simulink model "Simulink_Test_Model"  (R2018a)
settings: Solver=ode15s  StartTime=0.0  StopTime=100  FixedStep=0.0001  RelTol=1e-3  EnableMultiTasking=on
libraries: simulink x1
settings Model: Creator=user  LastModifiedBy=user
settings SolverCC: ConcurrentTasks=on  AutoInsertRateTranBlk=on
settings DataIOCC: SaveFormat=StructureWithTime  SaveState=on  SignalLoggingName=logsOut
settings OptimizationCC: BlockReduction=off  BooleanDataType=off  OptimizeBlockIOStorage=off  BufferReuse=off  GlobalBufferReuse=off  ExpressionFolding=off  LocalBlockOutputs=off  InitFltsAndDblsToZero=on  OptimizeDataStoreBuffers=off  BusAssignmentInplaceUpdate=off
settings DebuggingCC: SaveWithParameterizedLinksMsg=none  UnderspecifiedInitializationDetection=Classic  MergeDetectMultiDrivingBlocksExec=none  CheckExecutionContextPreStartOutputMsg=on  CheckExecutionContextRuntimeOutputMsg=on  SignalResolutionControl=TryResolveAllWithWarning  SFUnexpectedBacktrackingDiag=warning  SFNoUnconditionalDefaultTransitionDiag=warning  SFExecutionAtInitializationDiag=none
settings HardwareCC: ProdBitPerPointer=32  ProdBitPerSizeT=32  ProdBitPerPtrDiffT=32  ProdLargestAtomicFloat=None  ProdWordSize=32  ProdLongLongMode=on  ProdHWDeviceType=Generic->32-bit x86 compatible
settings ModelReferenceCC: PropagateSignalLabelsOutOfModel=off
settings RTWCC: SystemTargetFile=slrt.tlc  TemplateMakefile=slrt_default_tmf  Description=Simulink Real-Time  CodeExecutionProfiling=on  RTWCompilerOptimization=on
settings CodeAppCC: StateflowObjectComments=on
settings SimulinkRealTimeCC: SupportVariableSizeSignals=on  RL32LogTETModifier=off  xPCConcurrentTasks=on
settings ConfigComp: CovMetricSettings=dw  CovHtmlReporting=on  CovSaveCumulativeToWorkspaceVar=on  CovSaveSingleToWorkspaceVar=on  CovExternalEMLEnable=off  CovSFcnEnable=off

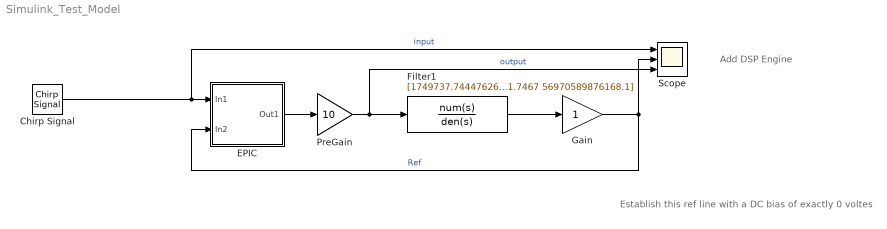
== system Simulink_Test_Model ==
  note: Establish this ref line with a DC bias of exactly 0 voltes
  note: Add DSP Engine
  Chirp Signal : simulink/Sources/Chirp Signal  f1=0.1  T=100  f2=100
  EPIC : Subsystem
  Filter1 : TransferFcn  Numerator=[1749737.74447626 456544220.2994 111217549558.059 15268939056263.4]  Denominator=[1 419038600.664162 35729810621.7467 56970589876168.1]
  Gain : Gain  SaturateOnIntegerOverflow=on  OutDataTypeStr=Inherit: Same as input  ParamDataTypeStr=Inherit: Same as input
  PreGain : Gain  Gain=10  OutMin=-5  OutMax=5  SaturateOnIntegerOverflow=on  OutDataTypeStr=Inherit: Same as input  ParamDataTypeStr=Inherit: Same as input
  Scope : Scope  NumInputPorts=3
  wires:
  Gain/1 -> EPIC/2(In2), Scope/2  "Ref"
  EPIC/1(Out1) -> PreGain/1
  Filter1/1 -> Gain/1
  Chirp Signal/1 -> Scope/1, EPIC/1(In1)  "input"
  PreGain/1 -> Filter1/1, Scope/3  "output"

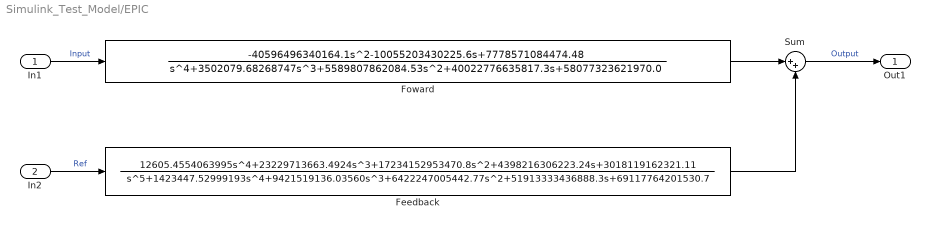
== system Simulink_Test_Model/EPIC ==
  In1 : Inport
  In2 : Inport  Port=2
  Feedback : TransferFcn  Numerator=[12605.4554063995,23229713663.4924,17234152953470.8,4398216306223.24,3018119162321.11]  Denominator=[1,1423447.52999193,9421519136.03560,6422247005442.77,51913333436888.3,69117764201530.7]
  Foward : TransferFcn  Numerator=[-40596496340164.1,-10055203430225.6,7778571084474.48]  Denominator=[1,3502079.68268747,5589807862084.53,40022776635817.3,58077323621970.0]
  Sum : Sum  Inputs=|++  OutMin=[-100]  OutMax=[100]
  Out1 : Outport
  wires:
  In1/1 -> Foward/1  "Input"
  Sum/1 -> Out1/1  "Output"
  In2/1 -> Feedback/1  "Ref"
  Foward/1 -> Sum/1
  Feedback/1 -> Sum/2
